simulink model "hw1_demo"  (R2025a)
settings: Solver=VariableStepAuto  StartTime=0.0  StopTime=10.0  RelTol=1e-3
settings Model: Creator=LEGION  LastModifiedBy=LEGION

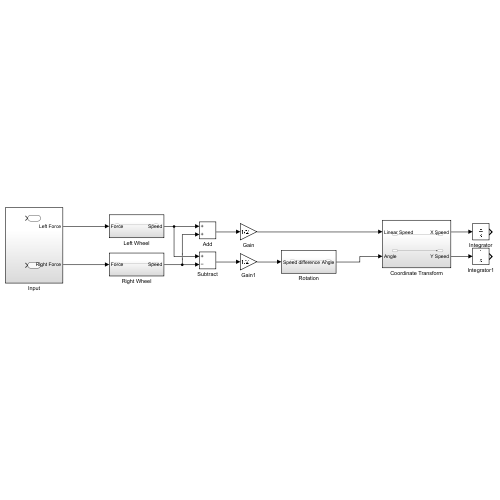
[thumbnail: Simulink's stored preview of the top-level diagram]
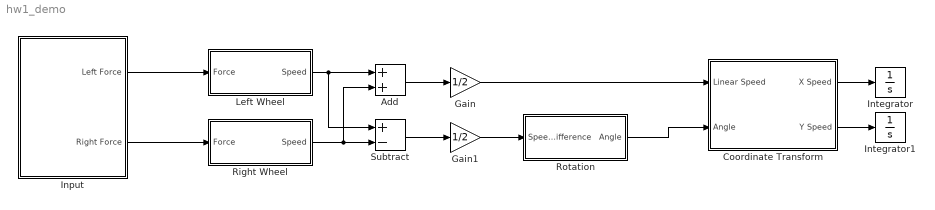
== system hw1_demo ==
  Add : Sum
  Coordinate Transform : Subsystem
  Gain : Gain  Gain=1/2
  Gain1 : Gain  Gain=1/2
  Input : Subsystem
  Integrator : Integrator
  Integrator1 : Integrator
  Left Wheel : Subsystem
  Right Wheel : Subsystem
  Rotation : Subsystem
  Subtract : Sum  Inputs=+-
  wires:
  Input/1(Left Force) -> Left Wheel/1(Force)
  Input/2(Right Force) -> Right Wheel/1(Force)
  Right Wheel/1(Speed) -> Subtract/2, Add/2
  Left Wheel/1(Speed) -> Add/1, Subtract/1
  Add/1 -> Gain/1
  Subtract/1 -> Gain1/1
  Gain/1 -> Coordinate Transform/1(Linear Speed)
  Gain1/1 -> Rotation/1(Speed difference)
  Rotation/1(Angle) -> Coordinate Transform/2(Angle)
  Coordinate Transform/1(X Speed) -> Integrator/1
  Coordinate Transform/2(Y Speed) -> Integrator1/1

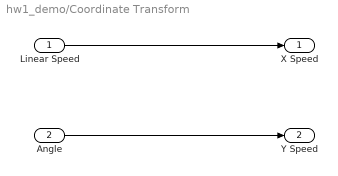
== system hw1_demo/Coordinate Transform ==
  Linear Speed : Inport
  Angle : Inport  Port=2
  X Speed : Outport
  Y Speed : Outport  Port=2
  wires:
  Linear Speed/1 -> X Speed/1
  Angle/1 -> Y Speed/1

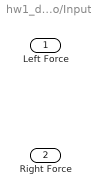
== system hw1_demo/Input ==
  Left Force : Outport
  Right Force : Outport  Port=2

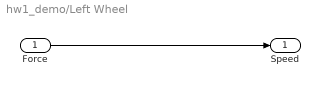
== system hw1_demo/Left Wheel ==
  Force : Inport
  Speed : Outport
  wires:
  Force/1 -> Speed/1

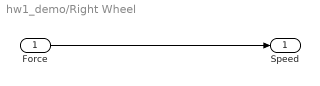
== system hw1_demo/Right Wheel ==
  Force : Inport
  Speed : Outport
  wires:
  Force/1 -> Speed/1

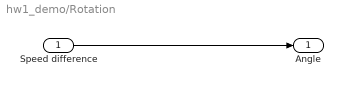
== system hw1_demo/Rotation ==
  Speed difference : Inport
  Angle : Outport
  wires:
  Speed difference/1 -> Angle/1
